simulink model "fSystemRLIM"  (R2025b)
settings: Solver=VariableStepAuto  StartTime=0.0  StopTime=0.1  RelTol=1e-3
libraries: rllib x1
settings Model: Creator=yilee  LastModifiedBy=joshu
settings OptimizationCC: ReuseModelBlockBuffer=off
settings RTWCC: GPUComputeCapability=3.5

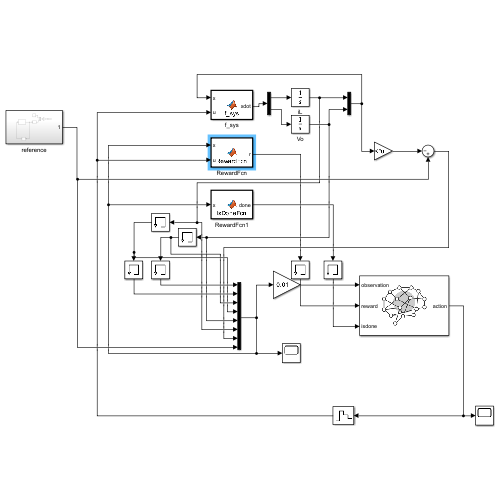
[thumbnail: Simulink's stored preview of the top-level diagram]
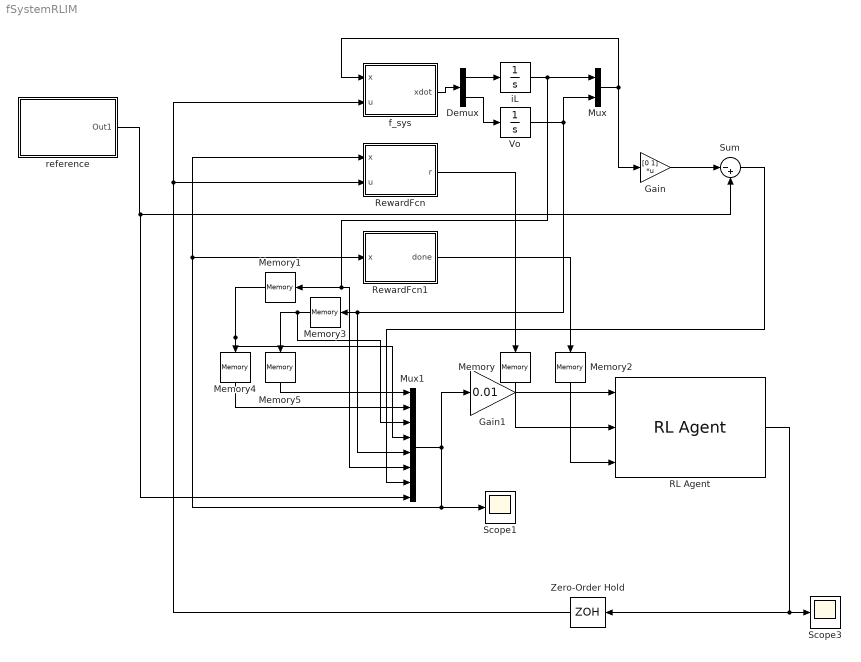
== system fSystemRLIM ==
  Demux : Demux  Outputs=2
  Gain : Gain  Gain=[0 1]  Multiplication=Matrix(K*u)
  Gain1 : Gain  Gain=0.01
  Memory{,1..5} (6 alike) : Memory  InheritSampleTime=on
  Mux : Mux  Inputs=2
  Mux1 : Mux  Inputs=8
  RL Agent : rllib/RL Agent  Agent=bestAgent  ExternalActionAsInput=off  ProvideLastAction=off  ProvideCumRwd=off  TreatAsDirectFeedthrough=on  UseStrictObservationDataTypes=off
  RewardFcn : MATLAB Function  TreatAsAtomicUnit=on
  RewardFcn1 : MATLAB Function  TreatAsAtomicUnit=on
  Scope1 : Scope
      settings: TimeSpan=0.1  ActiveDisplayYMinimum=-200  ActiveDisplayYMaximum=200
  Scope3 : Scope
      settings: TimeSpan=0.1  ActiveDisplayYMinimum=-1.3196723336783704  ActiveDisplayYMaximum=0.58501865942928855  DataLoggingVariableName=ScopeData2
  Sum : Sum  Inputs=|-+
  Vo : Integrator
  Zero-Order Hold : ZeroOrderHold  SampleTime=200e-6
  f_sys : MATLAB Function  TreatAsAtomicUnit=on
  iL : Integrator
  reference : Subsystem
  wires:
  Mux/1 -> f_sys/1(x), Gain/1
  RewardFcn/1(r) -> Memory/1
  RewardFcn1/1(done) -> Memory2/1
  Memory/1 -> RL Agent/2
  Memory2/1 -> RL Agent/3
  Zero-Order Hold/1 -> f_sys/2(u), RewardFcn/2(u)
  Gain/1 -> Sum/1
  Mux1/1 -> Gain1/1, Scope1/1, RewardFcn1/1(x), RewardFcn/1(x)
  f_sys/1(xdot) -> Demux/1
  Demux/1 -> iL/1
  Demux/2 -> Vo/1
  iL/1 -> Memory1/1, Mux1/6, Mux/1
  Vo/1 -> Mux1/5, Memory3/1, Mux/2
  RL Agent/1 -> Zero-Order Hold/1, Scope3/1
  Gain1/1 -> RL Agent/1
  Memory3/1 -> Mux1/3, Memory5/1
  Memory1/1 -> Mux1/4, Memory4/1
  Memory5/1 -> Mux1/1
  Memory4/1 -> Mux1/2
  Sum/1 -> Mux1/7
  reference/1(Out1) -> Mux1/8, Sum/2

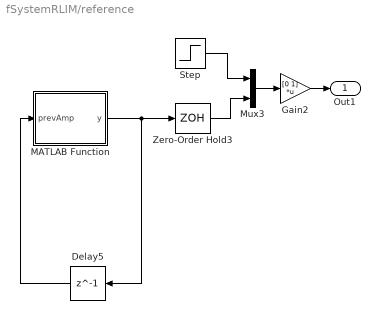
== system fSystemRLIM/reference ==
  Delay5 : Delay  DelayLength=1  SampleTime=200e-6
  Gain2 : Gain  Gain=[0 1]  Multiplication=Matrix(K*u)
  MATLAB Function : MATLAB Function  TreatAsAtomicUnit=on  SystemSampleTime=0.02
  Mux3 : Mux  Inputs=2
  Step : Step  Time=0.05  Before=45  After=55  SampleTime=0
  Zero-Order Hold3 : ZeroOrderHold  SampleTime=200e-6
  Out1 : Outport
  wires:
  MATLAB Function/1(y) -> Zero-Order Hold3/1, Delay5/1
  Mux3/1 -> Gain2/1
  Delay5/1 -> MATLAB Function/1(prevAmp)
  Zero-Order Hold3/1 -> Mux3/2
  Gain2/1 -> Out1/1
  Step/1 -> Mux3/1

== matlab function fSystemRLIM/f_sys ==
  data: x input size=[2 1]; u input size=[1 1]; xdot output
function xdot = f_sys(x,u)
%#codegen
    % 파라미터 정의
    R = 500;
    L = 840e-6; 
    C = 4.7e-3; 
    vi = 100;    
    Pcpl = 0;  

    % 1. 입력 u 안전장치 (0~1 범위 자르기)
    % 에이전트가 -1~1을 주더라도 0~1로 변환해서 써야 합니다.
    % (만약 Simulink 밖에서 이미 변환했다면 u를 그대로 써도 됨)
    u_safe = (u + 1) / 2;       % -1~1 -> 0~1 변환
    u_safe = max(0, min(1, u_safe)); 

    % 상태 변수
    iL = x(1);
    vo = x(2);
    
    if abs(vo) < 1e-6
        i_cpl = 0; % 전압이 0에 가까우면 부하 전류도 0으로 간주
    else
        i_cpl = Pcpl / vo;
    end
    
    
    % 3. 미분 방정식
    x1_dot = -1/L * vo + (vi/L * u_safe); 
    x2_dot = (iL - i_cpl - vo/R) / C;
    
    xdot = [x1_dot; x2_dot];
end

== matlab function fSystemRLIM/RewardFcn1 ==
  data: x input; done output
function done = IsDoneFcn(x)
% 상태 어느 성분이든 |xi| > xmax 이면 종료
    xmax = 100000;
    if any(abs(x) > xmax)
        done = true;
    else
        done = false;
    end
%    done=false;
end

== matlab function fSystemRLIM/reference/MATLAB Function ==
  data: y output; prevAmp input
function y = randomStep(prevAmp)
%#codegen
% t: 현재 시간
% prevAmp: 이전 스텝에서의 amplitude (Unit Delay 출력)
%
% 출력: random amplitude 또는 0

    % 첫 실행 시 prevAmp = 0으로 오므로 새 랜덤 생성
    if prevAmp == 0
        rng('shuffle','twister');
        amp = 40 + rand * (60 - 40);   % Simulink에서 rand() 가능
    else
        amp = prevAmp;
    end
    y=amp;
end

== matlab function fSystemRLIM/RewardFcn ==
  data: x input; u input; r output
function r = RewardFcn(x,u)
%#codegen
% x(5): iL (인덕터 전류)
% x(6): vo (출력 전압)
% x(7): Voltage Error (Vref - vo)

    %% 1. 파라미터 및 최대값 정의 (시스템 환경에 맞게 수정 필요)
    
    % **정규화 기준 값 (사용자 시스템의 최대/목표 값으로 설정하세요)**
    I_L_MAX   = 30.0;     % 인덕터 전류의 예상 최대값 (예: 30A)
    V_ERR_MAX = 60.0;     % 전압 에러의 예상 최대값 (Max Vref - Min Vo)
    I_L_LIMIT = 24.0;     % 인덕터 전류 제한 값 (논문 sigma)
    
    % 보상 함수 계수 (음수 값은 페널티, 양수 값은 보너스)
    ALPHA_VOL = 0.5;      % 전압 페널티 강도 (클수록 에러에 민감)
    GAMMA_CUR = 1;     % 전류 오버슛 페널티 강도 (매우 강하게)
    
    %% 2. 상태 정규화 및 에러 정의
    
    % 전압 에러 정규화: |Vref - vo| / V_ERR_MAX (0 ~ 1.0 범위)
    v_error_abs = abs(x(7));
    v_error_norm = v_error_abs / V_ERR_MAX; 
    
    % 전류 절대값 정규화: |iL| / I_L_MAX
    i_L_abs = abs(x(5));
    i_L_norm = i_L_abs / I_L_MAX; 
    
    %% 3. 전압 보상 (r_vol) - 이차 페널티 (Quadratic Penalty)
    
    r_vol = -ALPHA_VOL * (v_error_norm^2); 
    
    %% 4. 전류 보상 (r_cur) - Soft Penalty
    
    if i_L_abs >= I_L_LIMIT
        % 전류 제한(24A)을 넘으면 강력한 페널티 (오버슛 부분의 제곱에 비례)
        % 이 페널티는 전압 보상보다 강해야 합니다 (제한 조건이므로).
        i_overshoot_norm = (i_L_abs - I_L_LIMIT) / I_L_MAX; % 오버슛 부분만 정규화
        r_cur = -GAMMA_CUR * (i_overshoot_norm^2);
    else
        r_cur = 0;
    end
    
    %% 5. 최종 보상 합산 및 스케일링
    % 최종 보상 r은 대략 -10 ~ +1.0 사이의 안정적인 값으로 형성됩니다.
    r = r_vol + r_cur;
    
end
